simulink model "chap4_4sim"  (Simulink 8.3)
settings: Solver=ode45  StartTime=0.0  StopTime=100  RelTol=1e-3
settings Model: Creator=liujk  LastModifiedBy=Administrator  ExtModeTrigMode=oneshot  ExtModeArmWhenConnect=off
settings DataIOCC: LimitDataPoints=off
settings OptimizationCC: BlockReduction=off  BooleanDataType=off
settings DebuggingCC: SaveWithParameterizedLinksMsg=none  SignalResolutionControl=TryResolveAllWithWarning  SolverPrmCheckMsg=none  MultiTaskDSMMsg=warning  MultiTaskCondExecSysMsg=none
settings HardwareCC: TargetUnknown=on
settings RTWCC: IncludeERTFirstTime=on

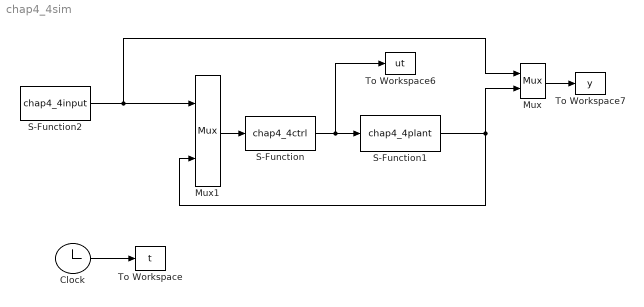
== system chap4_4sim ==
  Clock : Clock
  Mux : Mux  Inputs=2
  Mux1 : Mux  Inputs=2
  S-Function : S-Function  FunctionName=chap4_4ctrl  EnableBusSupport=off
  S-Function1 : S-Function  FunctionName=chap4_4plant  EnableBusSupport=off
  S-Function2 : S-Function  FunctionName=chap4_4input  EnableBusSupport=off
  To Workspace : ToWorkspace  VariableName=t  SampleTime=-1
  To Workspace6 : ToWorkspace  VariableName=ut  SampleTime=-1
  To Workspace7 : ToWorkspace  VariableName=y  SampleTime=-1
  wires:
  Mux1/1 -> S-Function/1
  Mux/1 -> To Workspace7/1
  S-Function/1 -> S-Function1/1, To Workspace6/1
  Clock/1 -> To Workspace/1
  S-Function2/1 -> Mux/1, Mux1/1
  S-Function1/1 -> Mux1/2, Mux/2
